simulink model "blobDetect"  (R2013b)
settings: Solver=FixedStepDiscrete  StartTime=0.0  StopTime=inf  RelTol=1e-3
PreLoadFcn:
  | load projectionMatrix.mat
undefined symbols (not defined in the file or in its folder): delay, IsPositionTracked, IsSkeletonTracked, jet, JointDepthIndices, JointImageIndices, JointTrackingState, JointWorldCoordinates, magnitude, none, PositionDepthIndices, PositionImageIndices, PositionWorldCoordinates, Rec, SDTV, SegmentationData, SkeletonTrackingID, videoinput
libraries: dspindex x3, visionstatistics x2, simulink x2, visionsinks x2, visionconversions x1, visionanalysis x1, dspbuff3 x1, visiontextngfix x1, imaqlib x1
settings Model: Creator=vleung  LastModifiedBy=vleung
settings OptimizationCC: ExpressionDepthLimit=2147483647
settings DebuggingCC: StateNameClashWarn=warning

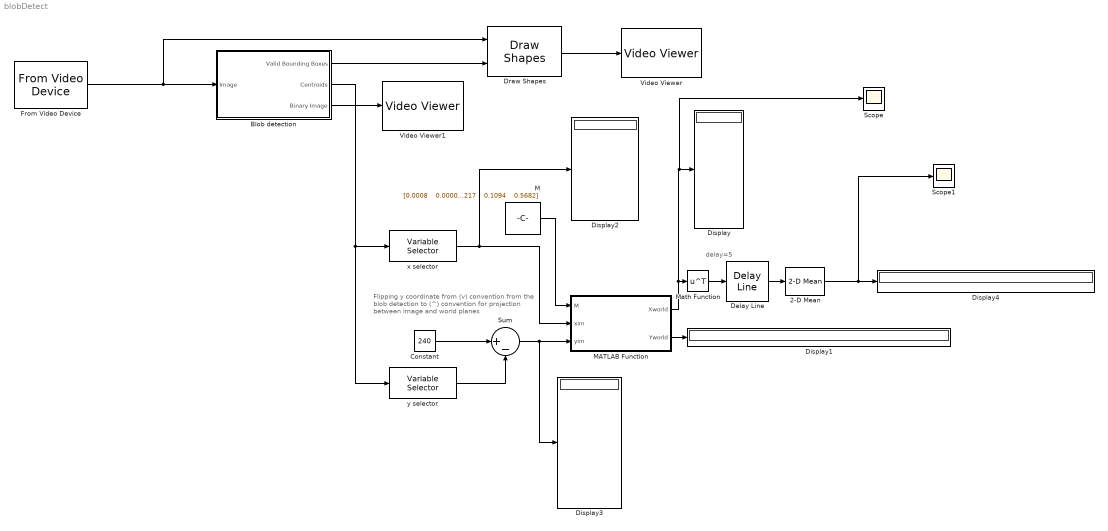
== system blobDetect ==
  note: delay=5
  note: Flipping y coordinate from (v) convention from
      | the blob detection to (^) convention for projection
      | between image and world planes
  2-D Mean : visionstatistics/2-D Mean  run=off  reset_popup=None  directionMode=Each column  dimension=1  treatSBRowAsCol=on  roiEnable=off  roiType=Rectangles  roiPortion=Entire ROI  roiOutput=Individual statistics for each ROI  roiFlag=off  outputDataTypeStr=Inherit: Same as accumulator  outputLastDataTypeStr=Inherit: Same as accumulator  outputMin=[]  outputMax=[]  accumMode=Binary point scaling  accumWordLength=32  accumFracLength=0  accumDataTypeStr=fixdt([],32,0)  accumLastDataTypeStr=fixdt([],32,0)  roundingMode=Floor  overflowMode=off
  Blob detection : Subsystem
  Constant : Constant  Value=240
  Delay Line : dspbuff3/Delay Line  siz=6*delay  ic=0  directfeed=off  enable_output=off  hold_output=off  TreatMby1Signals=One channel
  Display{,1..4} (5 alike) : Display
  Draw Shapes : visiontextngfix/Draw Shapes  shape=Rectangles  fill=off  fillClrSource=Specify via dialog  display=User-specified value  intensity=200  color=[0 0 0]  opacity=0.6  viewport=Entire image  antialiasing=off  inType=Obsolete  imagePorts=One multidimensional signal  prodOutputMode=Binary point scaling  prodOutputWordLength=32  prodOutputFracLength=14  memoryMode=Specify word length  memoryWordLength=16  memoryFracLength=15  roundingMode=Floor  overflowMode=off
  From Video Device : imaqlib/From Video Device  DeviceMenu=mwdemoimaq 1 (Color Device)  Device=winvideo 1 (Microsoft LifeCam Cinema)  ObjConstructor=videoinput('winvideo', 1)  VideoFormatMenu=RGB_NTSC  VideoFormat=MJPG_320x240  VideoSource=input1  ROIPosition=[0 0 240 320]  EnableHWTrigger=off  TriggerConfiguration=none/none  SampleTime=1/30  OutputPortsMode=One multidimensional signal  DataType=single  CanDoHWTrigger=no  ReturnedColorSpace=rgb  BlockHandle=2.0043  ROIWidth=320  ROIHeight=240  ROIColumn=0  ROIRow=0  EngXMLPath=C:\Program Files\MATLAB\R2013b_64bit\toolbox\imaq\imaq\private  DevXMLPath=C:\Program Files\MATLAB\R2013b_64bit\toolbox\imaq\imaqadaptors\win64  EngLibPath=C:\Program Files\MATLAB\R2013b_64bit\toolbox\imaq\imaqblks\imaqmex\win64  ColorSpace=rgb  BayerSensorAlignment=grbg  AllMetadata=IsPositionTracked;IsSkeletonTracked;JointDepthIndices;JointImageIndices;JointTrackingState;JointWorldCoordinates;PositionDepthIndices;PositionImageIndices;PositionWorldCoordinates;SegmentationData;SkeletonTrackingID
  M : Constant  Value="[0.0008    0.0000   -0.0000; 0.0000    0.0004   -0.0016; -0.1217    0.1094    0.5682]"  VectorParams1D=off
  MATLAB Function : MATLAB Function  TreatAsAtomicUnit=on
  Math Function : Math  Operator=transpose  SaturateOnIntegerOverflow=on
  Scope : Scope
      settings: YMin=-0.7  YMax=0.3
  Scope1 : Scope
      settings: YMin=-0.7  YMax=0.3
  Sum : Sum  Inputs=|+-
  Video Viewer : visionsinks/Video Viewer  inputType=Obsolete7b  imagePorts=One multidimensional signal  useColorMap=off  colormapValue=jet(256)  specRange=off  minInputVal=0  maxInputVal=255  FigPos=[32 700 578 357]  AxisZoom=on  trueSizedOnce=off  OpenAtMdlStart=on  DefaultConfigurationName=vipscopes.VideoViewerScopeCfg
  Video Viewer1 : visionsinks/Video Viewer  inputType=Obsolete7b  imagePorts=One multidimensional signal  useColorMap=off  colormapValue=jet(256)  specRange=off  minInputVal=0  maxInputVal=255  FigPos=[89 1091 410 300]  AxisZoom=on  trueSizedOnce=off  OpenAtMdlStart=on  DefaultConfigurationName=vipscopes.VideoViewerScopeCfg
  x selector : dspindex/Variable Selector  NumInputs=1  rowsOrCols=Columns  IdxMode=Fixed  Elements=1  ZerOneIdxMode=One-based  errmode=Generate Error  FillMode=on  FillValues=0
  y selector : dspindex/Variable Selector  NumInputs=1  rowsOrCols=Columns  IdxMode=Fixed  Elements=2  ZerOneIdxMode=One-based  errmode=Generate Error  FillMode=on  FillValues=0
  wires:
  Draw Shapes/1 -> Video Viewer/1
  From Video Device/1 -> Draw Shapes/1, Blob detection/1(Image)
  Blob detection/3(Binary Image) -> Video Viewer1/1
  Blob detection/1(Valid Bounding Boxes) -> Draw Shapes/2
  Blob detection/2(Centroids) -> y selector/1, x selector/1
  y selector/1 -> Sum/2
  Constant/1 -> Sum/1
  Sum/1 -> Display3/1, MATLAB Function/3(yim)
  x selector/1 -> Display2/1, MATLAB Function/2(xim)
  MATLAB Function/1(Xworld) -> Math Function/1, Scope/1, Display/1
  MATLAB Function/2(Yworld) -> Display1/1
  M/1 -> MATLAB Function/1(M)
  Delay Line/1 -> 2-D Mean/1
  2-D Mean/1 -> Scope1/1, Display4/1
  Math Function/1 -> Delay Line/1

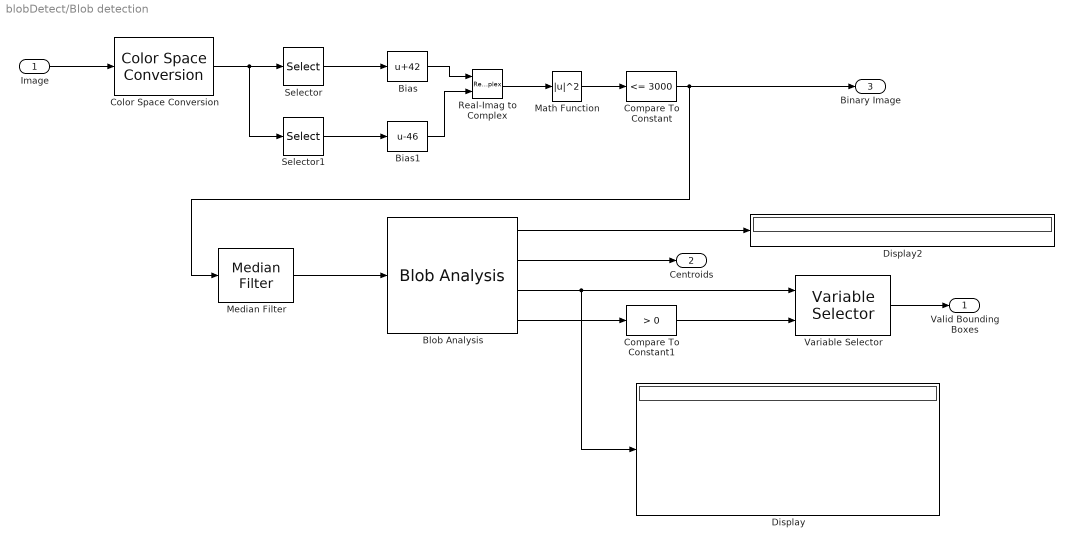
== system blobDetect/Blob detection ==
  Image : Inport
  Bias : Bias  Bias=42
  Bias1 : Bias  Bias=-46
  Blob Analysis : visionstatistics/Blob Analysis  Tag=vipblks_row_conv  area=on  centroid=on  bBox=on  majorAxis=off  minorAxis=off  angle=off  eccentricity=on  equivDiameterSq=off  extent=off  perimeter=off  maxBlobs=6  warnIfNumBlobsExceeded=off  isCount=off  useMinArea=on  minArea=50  useMaxArea=off  maxArea=intmax('uint32')  excludeBorderBlob=on  outDT=double  isOutVarDim=off  isFill=on  fillValues=-1  conn=8  isLabel=off  outputMode=Binary point scaling  outputWordLength=32  outputFracLength=16  firstCoeffMode=Binary point scaling  firstCoeffWordLength=16  firstCoeffFracLength=14  secondCoeffMode=Binary point scaling  secondCoeffWordLength=32  secondCoeffFracLength=16  accumMode=Binary point scaling  accumWordLength=32  accumFracLength=0  prodOutputMode=Binary point scaling  prodOutputWordLength=32  prodOutputFracLength=16  roundingMode=Floor  overflowMode=off
  Color Space Conversion : visionconversions/Color Space  Conversion  conversion=Obsolete  conversionActive=sR'G'B' to L*a*b*  wp_str=D65  rec=Rec. 601 (SDTV)  sys=1125/60/2:1  imagePorts=One multidimensional signal
  Compare To Constant : simulink/Logic and Bit Operations/Compare To Constant  relop=<=  const=3000  OutDataTypeStr=boolean
  Compare To Constant1 : simulink/Logic and Bit Operations/Compare To Constant  relop=>  const=0  OutDataTypeStr=boolean
  Display : Display
  Display2 : Display
  Math Function : Math  Operator=magnitude^2  SaturateOnIntegerOverflow=on
  Median Filter : visionanalysis/Median Filter  nghbood=[3 3]  outSize=Same as input port I  padType=Constant  padSrc=Specify via dialog  padVal=0  roundingMode=Floor  overflowMode=off
  Real-Imag to Complex : RealImagToComplex
  Selector : Selector  NumberOfDimensions=3  InputPortWidth=3  IndexOptions=Select all,Select all,Index vector (dialog)  Indices=[1 3],1,2  OutputSizes=1,1,1
  Selector1 : Selector  NumberOfDimensions=3  InputPortWidth=3  IndexOptions=Select all,Select all,Index vector (dialog)  Indices=[1 3],1,3  OutputSizes=1,1,1
  Variable Selector : dspindex/Variable Selector  NumInputs=1  rowsOrCols=Rows  IdxMode=Variable  Elements=[1 3]  ZerOneIdxMode=One-based  errmode=Generate Error  FillMode=on  FillValues=0
  Valid Bounding Boxes : Outport
  Centroids : Outport  Port=2
  Binary Image : Outport  Port=3
  wires:
  Bias/1 -> Real-Imag to Complex/1
  Real-Imag to Complex/1 -> Math Function/1
  Median Filter/1 -> Blob Analysis/1
  Math Function/1 -> Compare To Constant/1
  Image/1 -> Color Space Conversion/1
  Color Space Conversion/1 -> Selector1/1, Selector/1
  Compare To Constant1/1 -> Variable Selector/2
  Blob Analysis/4 -> Compare To Constant1/1
  Compare To Constant/1 -> Binary Image/1, Median Filter/1
  Bias1/1 -> Real-Imag to Complex/2
  Blob Analysis/3 -> Variable Selector/1, Display/1
  Selector/1 -> Bias/1
  Variable Selector/1 -> Valid Bounding Boxes/1
  Selector1/1 -> Bias1/1
  Blob Analysis/2 -> Centroids/1
  Blob Analysis/1 -> Display2/1

== matlab function blobDetect/MATLAB Function ==
  data: M input; Xworld output; xim input; yim input; Yworld output
function [Xworld, Yworld] = image2world(M, xim, yim)
%#codegen

% Inputs: xim = [nx1] vector of x-coordinate in image plane
%         yim = [nx1] vector of y-coordinate in image plane
%         
%         For the image coordinates, origin is bottom left, convention:
%         x (>), y(^)
%
% Outputs: Xworld = [nx1] vector of x-coordinates in world plane
%          Yworld = [nx1] vector of y-coordinates in world plane
%          
%          For the world coordinates, robot at (X,Y) = (0,0)
%

if size(xim, 2) > size(xim, 1)
    xim = xim' ;
end

if size(yim, 2) > size(yim, 1)
    yim = yim' ;
end
    
% [Xworld,Yworld] = transformPointsInverse(t_world2im, xim, yim) ;
% transformPointsInverse does not support codegen, but can get code from
% its class projective2d.

% M = inv( t_world2im );
u = M(1,1).*xim + M(2,1).*yim + M(3,1);
v = M(1,2).*xim + M(2,2).*yim + M(3,2);
w = M(1,3).*xim + M(2,3).*yim + M(3,3);

Xworld = u./w ;
Yworld = v./w ;

% limite the minimum Yworld to 0
Yworld = max([Yworld, zeros(size(Yworld))],[],2) ;
